simulink model "project_1"  (R2023a)
settings: Solver=ode45  StartTime=0.0  StopTime=10.0  MaxStep=0.01  RelTol=1e-3
settings Model: Creator=FC  LastModifiedBy=FC

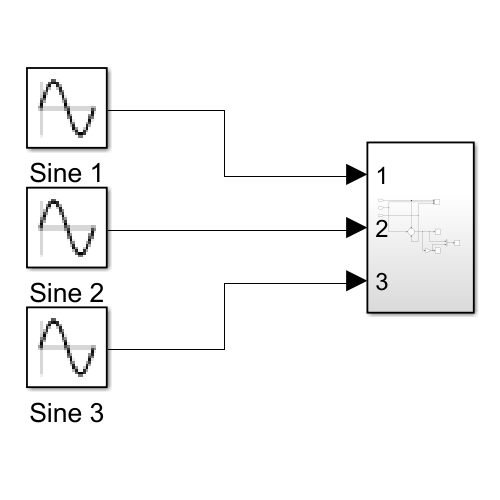
[thumbnail: Simulink's stored preview of the top-level diagram]
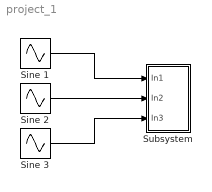
== system project_1 ==
  Sine 1 : Sin  SampleTime=0
  Sine 2 : Sin  Frequency=5  SampleTime=0
  Sine 3 : Sin  Frequency=7  SampleTime=0
  Subsystem : Subsystem
  wires:
  Sine 1/1 -> Subsystem/1(In1)
  Sine 2/1 -> Subsystem/2(In2)
  Sine 3/1 -> Subsystem/3(In3)

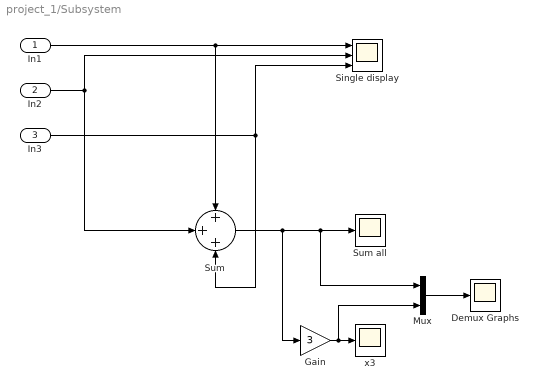
== system project_1/Subsystem ==
  In1 : Inport
  In2 : Inport  Port=2
  In3 : Inport  Port=3
  Demux Graphs : Scope
  Gain : Gain  Gain=3
  Mux : Mux  Inputs=2
  Single display : Scope  NumInputPorts=3
  Sum : Sum  Inputs=+++
  Sum all : Scope
  x3 : Scope
  wires:
  Mux/1 -> Demux Graphs/1
  Gain/1 -> Mux/2, x3/1
  In1/1 -> Sum/1, Single display/1
  Sum/1 -> Gain/1, Mux/1, Sum all/1
  In2/1 -> Sum/2, Single display/2
  In3/1 -> Sum/3, Single display/3
